simulink model "dummy_syst"  (R2020b)
settings: Solver=VariableStepAuto  StartTime=0.0  StopTime=10.0  RelTol=1e-3
settings Model: Creator=Martin  LastModifiedBy=Martin

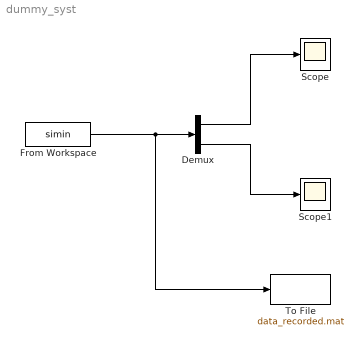
== system dummy_syst ==
  Demux : Demux  Outputs=2
  From Workspace : FromWorkspace  VariableName=simin
  Scope : Scope
  Scope1 : Scope
  To File : ToFile  Filename=data_recorded.mat
  wires:
  From Workspace/1 -> To File/1, Demux/1
  Demux/1 -> Scope/1
  Demux/2 -> Scope1/1
